simulink model "DiodeRectifier_17b"  (R2020a)
settings: Solver=ode23tb  StartTime=0.0  StopTime=0.5  MaxStep=1e-4  RelTol=1e-3
libraries: powerlib x20, powerlib_meascontrol x7
settings Model: Creator=root  LastModifiedBy=Theodore
settings DataIOCC: ReturnWorkspaceOutputs=off
settings DebuggingCC: ArithmeticOperatorsInVariantConditions=warning
settings SFSimCC: SimUseLocalCustomCode=off  CustomCodeUndefinedFunction=UseInterfaceOnly
settings RTWCC: RTWUseLocalCustomCode=off
settings CodeAppCC: StateflowObjectComments=on
settings SimscapeCC: SimscapeNormalizeSystem=off

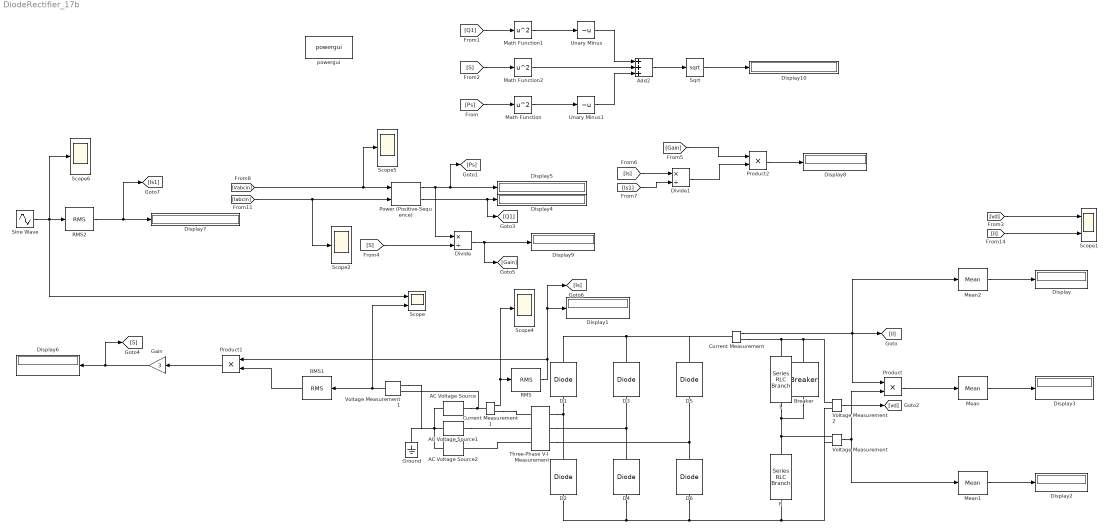
== system DiodeRectifier_17b ==
  AC Voltage Source : powerlib/Electrical Sources/AC Voltage Source  Amplitude=230*sqrt(2)  Phase=0  Frequency=50  SampleTime=0  Measurements=None  BusType=swing  Pref=10e3  Qref=0  Qmin=-inf  Qmax=+inf
  AC Voltage Source1 : powerlib/Electrical Sources/AC Voltage Source  Amplitude=230*sqrt(2)  Phase=-120  Frequency=50  SampleTime=0  Measurements=None  BusType=swing  Pref=10e3  Qref=0  Qmin=-inf  Qmax=+inf
  AC Voltage Source2 : powerlib/Electrical Sources/AC Voltage Source  Amplitude=230*sqrt(2)  Phase=120  Frequency=50  SampleTime=0  Measurements=None  BusType=swing  Pref=10e3  Qref=0  Qmin=-inf  Qmax=+inf
  Add2 : Sum  Inputs=+++
  Breaker : powerlib/Elements/Breaker  InitialState=0  SwitchingTimes="[2  20]"  External=off  BreakerResistance=0.01  SnubberResistance=1e6  SnubberCapacitance=inf  Measurements=None  MoreParameters=on  NoBreakLoop=off
  Current Measurement : powerlib/Measurements/Current Measurement  PhasorSimulation=off  OutputType=Complex  PSBequivalent=0
  Current Measurement1 : powerlib/Measurements/Current Measurement  PhasorSimulation=off  OutputType=Complex  PSBequivalent=0
  D{1..6} (6 alike) : powerlib/Power Electronics/Diode  Ron=0.001  Lon=0  Vf=0.8  IC=0  UseSnubber=0  Rs=500  Cs=250e-9  Measurements=off
  Display{,1..10} (11 alike) : Display
  Divide : Product  Inputs=*/
  Divide1 : Product  Inputs=*/
  Gain : Gain  Gain=3
  Ground : powerlib/Elements/Ground  LConnTagsString=a
  L : powerlib/Elements/Series RLC Branch  LConnTagsString=__new0  RConnTagsString=__new0  BranchType=L  Resistance=1  Inductance=0.0000001  SetiL0=off  InitialCurrent=0  Capacitance=1e-6  Setx0=off  InitialVoltage=0  Measurements=None
  Math Function : Math  Operator=square  SaturateOnIntegerOverflow=on
  Math Function1 : Math  Operator=square  SaturateOnIntegerOverflow=on
  Math Function2 : Math  Operator=square  SaturateOnIntegerOverflow=on
  Mean : powerlib_meascontrol/Measurements/Mean  Freq=50  Vinit=0  Ts=0
  Mean1 : powerlib_meascontrol/Measurements/Mean  Freq=50  Vinit=0  Ts=0
  Mean2 : powerlib_meascontrol/Measurements/Mean  Freq=50  Vinit=0  Ts=0
  Power (Positive-Sequence) : powerlib_meascontrol/Measurements/Power (Positive-Sequence)  Freq=50  Vinit=[0, 0]  Iinit=[0, 0]  Ts=0
      settings: SourceProductBaseCode=PS
  Product : Product
  Product1 : Product
  Product2 : Product
  R : powerlib/Elements/Series RLC Branch  LConnTagsString=__new0  RConnTagsString=__new0  BranchType=R  Resistance=50  Inductance=1e-3  SetiL0=off  InitialCurrent=0  Capacitance=1e-6  Setx0=off  InitialVoltage=0  Measurements=Branch current
  RMS : powerlib_meascontrol/Measurements/RMS  TrueRMS=on  Freq=50  RMSInit=120  Ts=0
  RMS1 : powerlib_meascontrol/Measurements/RMS  TrueRMS=on  Freq=50  RMSInit=120  Ts=0
  RMS2 : powerlib_meascontrol/Measurements/RMS  TrueRMS=on  Freq=50  RMSInit=120  Ts=0
  Scope : Scope  NumInputPorts=2
  Scope1 : Scope  NumInputPorts=2
  Scope{2,4..6} (4 alike) : Scope
  Sine Wave : Sin  Amplitude=11.88  Frequency=314.159265  Phase=-0.0745329252  SampleTime=0
  Sqrt : Sqrt  SaturateOnIntegerOverflow=on
  Three-Phase V-I Measurement : powerlib/Measurements/Three-Phase V-I Measurement  VoltageMeasurement=phase-to-ground  SetLabelV=on  LabelV=Vabcin  Vpu=off  VpuLL=off  CurrentMeasurement=yes  SetLabelI=on  LabelI=Iabcin  Ipu=off  Pbase=100e6  Vbase=500e3  OutputType=Complex  PhasorSimulation=off  PSBequivalent=0
  Unary Minus : UnaryMinus
  Unary Minus1 : UnaryMinus
  Voltage Measurement : powerlib/Measurements/Voltage Measurement  PhasorSimulation=off  OutputType=Complex  PSBequivalent=0
  Voltage Measurement1 : powerlib/Measurements/Voltage Measurement  PhasorSimulation=off  OutputType=Complex  PSBequivalent=0
  Voltage Measurement2 : powerlib/Measurements/Voltage Measurement  PhasorSimulation=off  OutputType=Complex  PSBequivalent=0
  powergui : powerlib/powergui  Priority=1  SimulationMode=Continuous  SampleTime=50e-6  frequency=60  Iterations=50  frequencyindice=50  Pbase=100e6  ErrMax=1e-4  UnitsV=kV  UnitsW=MW  buscounter=0  FunctionMessages=off  echomessages=off  EnableUseOfTLC=off  CurrentSourceSwitches=off  DisableSnubberDevices=on  DisableRonSwitches=on  DisableVfSwitches=on  DisplayEquations=off  AutomaticDiscreteSolvers=off  SolverType=Tustin/Backward Euler (TBE)  Interpol=off  ExternalGateDelay=off  methode=off  Ts=100  x0status=blocks  SPID=on  SwTol=0  HookPort=off  NonlinearTolerance=1e-4  nMaxIteration=100  ContinueOnMaxIteration=off  RestoreLinks=warning  ResistiveCurrentMeasurement=off  Frange=[0:2:500]  Ylog=off  Xlog=on  ShowGrid=off  save=off  variable=ZData  structure=Isa  ZoomFFT=off  StartTime=0.2  cycles=3  DisplayStyle=2  fundamental=50  FreqAxis=off  MaxFrequency=1000  frequencyindicesteady=1  RmsSteady=1  display=off
  wires:
  [vd] -> Scope1/1
  [il] -> Scope1/2
  [Iabcin] -> Scope2/1, Power (Positive-Sequence)/2
  [Vabcin] -> Scope5/1, Power (Positive-Sequence)/1
  Current Measurement/1 -> Mean2/1, [il], Product/1
  RMS/1 -> Display1/1, [Is], Product1/1
  Power (Positive-Sequence)/1 -> [Ps], Display5/1, Divide/1
  Power (Positive-Sequence)/2 -> [Q1], Display4/1
  Divide/1 -> [Gain], Display9/1
  [S] -> Math Function2/1
  [Ps] -> Math Function/1
  [Q1] -> Math Function1/1
  Math Function1/1 -> Unary Minus/1
  Math Function/1 -> Unary Minus1/1
  Unary Minus/1 -> Add2/1
  Unary Minus1/1 -> Add2/3
  Math Function2/1 -> Add2/2
  Add2/1 -> Sqrt/1
  Sqrt/1 -> Display10/1
  Voltage Measurement/1 -> Product/2, Mean1/1
  Product/1 -> Mean/1
  Mean/1 -> Display3/1
  Mean1/1 -> Display2/1
  Mean2/1 -> Display/1
  RMS1/1 -> Product1/2
  Voltage Measurement1/1 -> RMS1/1, Scope/2
  Product1/1 -> Gain/1
  Gain/1 -> Display6/1, [S]
  [S] -> Divide/2
  Current Measurement1/1 -> Scope4/1, RMS/1
  Sine Wave/1 -> Scope/1, Scope6/1, RMS2/1
  RMS2/1 -> [Is1], Display7/1
  [Gain] -> Product2/1
  Divide1/1 -> Product2/2
  Product2/1 -> Display8/1
  [Is] -> Divide1/1
  [Is1] -> Divide1/2
  Voltage Measurement2/1 -> [vd]
  connections:
  L/RConn1 -- Breaker/RConn1 -- Voltage Measurement/LConn1 -- R/LConn1
  D2/LConn1 -- D4/LConn1 -- Voltage Measurement2/LConn2 -- Voltage Measurement/LConn2 -- R/RConn1 -- D6/LConn1
  D4/RConn1 -- Three-Phase V-I Measurement/RConn2 -- D3/LConn1
  Three-Phase V-I Measurement/RConn3 -- D5/LConn1 -- D6/RConn1
  AC Voltage Source/RConn1 -- Voltage Measurement1/LConn1 -- Current Measurement1/LConn1
  D3/RConn1 -- D5/RConn1 -- Current Measurement/LConn1 -- D1/RConn1
  D1/LConn1 -- Three-Phase V-I Measurement/RConn1 -- D2/RConn1
  AC Voltage Source2/LConn1 -- Voltage Measurement1/LConn2 -- Ground/LConn1 -- AC Voltage Source1/LConn1 -- AC Voltage Source/LConn1
  Current Measurement1/RConn1 -- Three-Phase V-I Measurement/LConn1
  Breaker/LConn1 -- Voltage Measurement2/LConn1 -- Current Measurement/RConn1 -- L/LConn1
  Three-Phase V-I Measurement/LConn3 -- AC Voltage Source2/RConn1
  AC Voltage Source1/RConn1 -- Three-Phase V-I Measurement/LConn2
